simulink library "Feeder4_lib"  (Simulink 8.1)
settings: Solver=ode45  StartTime=0.0  StopTime=10.0  RelTol=1e-3
values from neighbouring files (symbols this model uses):
  DER_REL = xlsread('DER_relay.xlsx')    [relay_settings_init.m]
  Ts = 100E-6    (= 0.0001)    [BANSHEE_init.m]    (also in Ghost_init.m)
undefined symbols (not defined in the file or in its folder): CBID, Left, type, V
libraries: breaker_lib x9, Load_lib x7, cables_lib x3, relay_modbus_lib x3, rtio_generic_modbus x3, powerlib_meascontrol x3, NREL_Diesel_Genset_lib x2, BESS_lib x2, rtlab x2, simulink x2, ssn_lib x2, transformer_lib x1
settings Model: Creator=re25624  LastModifiedBy=MGC4

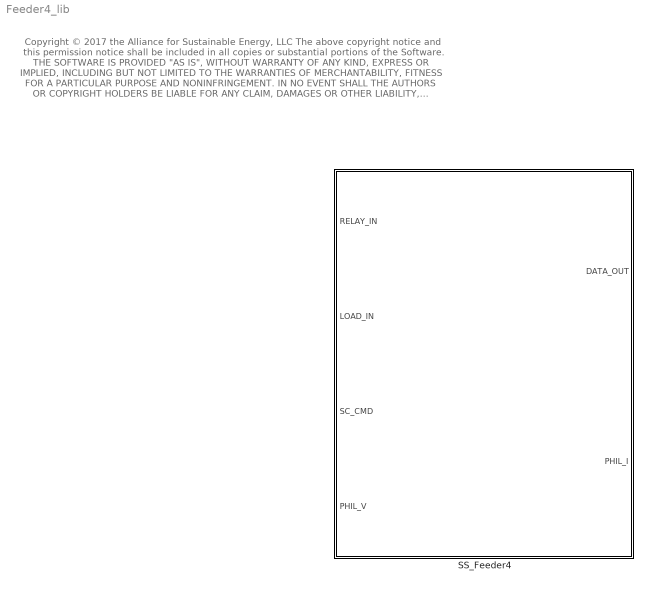
== system Feeder4_lib ==
  note: Copyright © 2017 the Alliance for Sustainable Energy, LLC
      |
      | The above copyright notice and this permission notice shall be included in all copies or substantial portions of the Software.
      |
      | THE SOFTWARE IS PROVIDED "AS IS", WITHOUT WARRANTY OF ANY KIND, EXPRESS OR IMPLIED, INCLUDING
      | BUT NOT LIMITED TO THE WARRANTIES OF MERCHANTABILITY, FITNESS FOR A PARTICULAR PURPOSE AND
      | NONINFRINGEMENT. IN NO EVENT SHALL THE AUTHORS OR COPYRIGHT HOLDERS BE LIABLE FOR ANY CLAIM,
      |  DAMAGES OR OTHER LIABILITY, WHETHER IN AN ACTION OF CONTRACT, TORT OR OTHERWISE, ARISING FROM,
      | OUT OF OR IN CONNECTION WITH THE SOFTWARE OR THE USE OR OTHER DEALINGS IN THE SOFTWARE
  SS_Feeder4 : Subsystem

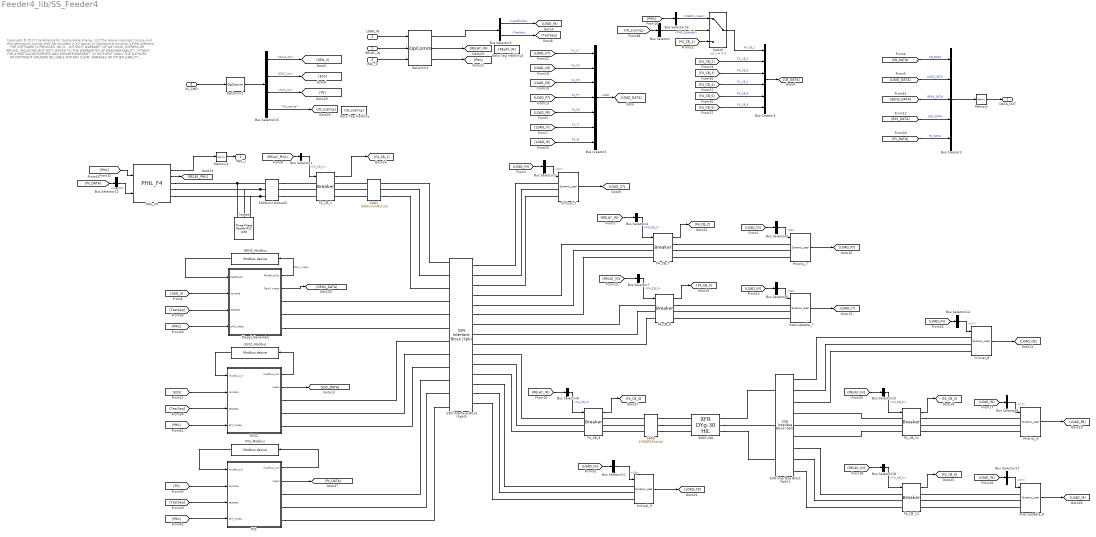
== system Feeder4_lib/SS_Feeder4 ==
  note: Copyright © 2017 the Alliance for Sustainable Energy, LLC
      |
      | The above copyright notice and this permission notice shall be included in all copies or substantial portions of the Software.
      |
      | THE SOFTWARE IS PROVIDED "AS IS", WITHOUT WARRANTY OF ANY KIND, EXPRESS OR IMPLIED, INCLUDING
      | BUT NOT LIMITED TO THE WARRANTIES OF MERCHANTABILITY, FITNESS FOR A PARTICULAR PURPOSE AND
      | NONINFRINGEMENT. IN NO EVENT SHALL THE AUTHORS OR COPYRIGHT HOLDERS BE LIABLE FOR ANY CLAIM,
      |  DAMAGES OR OTHER LIABILITY, WHETHER IN AN ACTION OF CONTRACT, TORT OR OTHERWISE, ARISING FROM,
      | OUT OF OR IN CONNECTION WITH THE SOFTWARE OR THE USE OR OTHER DEALINGS IN THE SOFTWARE
  RELAY_IN : Inport
  LOAD_IN : Inport  Port=2
  SC_CMD : Inport  Port=3
  PHIL_V : Inport  Port=4
  5000 kVA : transformer_lib/XFR DYg-30 HIL  Rating=50  Vp=480  Vs=208  Z=5.75  XR=4.7
  500kcmil-Mutual5 : cables_lib/500kcmil-Mutual  length=1000  par_sets=1  ratio=3
  Bus Creator2 : BusCreator  Inputs=5
  Bus Creator3 : BusCreator  Inputs=7
  Bus Creator5 : BusCreator  Inputs=6
  Bus Selector : BusSelector  OutputSignals=PHIL_Enabled
  Bus Selector1 : BusSelector  OutputSignals=F4_CB_1
  Bus Selector10 : BusSelector  OutputSignals=F4_CB_5
  Bus Selector11 : BusSelector  OutputSignals=C9
  Bus Selector12 : BusSelector  OutputSignals=pv_phil
  Bus Selector{2,9,14,17} (4 alike) : BusSelector  OutputSignals=C7
  Bus Selector15 : BusSelector  OutputSignals=Gen3_ctrl,ESS2_ctrl,PV2_ctrl,IO_scaling
  Bus Selector16 : BusSelector  OutputSignals=CB401_meas
  Bus Selector18 : BusSelector  OutputSignals=F4_CB_6
  Bus Selector3 : BusSelector  OutputSignals=C8
  Bus Selector4 : BusSelector  OutputSignals=F4_CB_2
  Bus Selector5 : BusSelector  OutputSignals=LoadProfile,TestSeq
  Bus Selector6 : BusSelector  OutputSignals=C8
  Bus Selector7 : BusSelector  OutputSignals=F4_CB_3
  Bus Selector8 : BusSelector  OutputSignals=F4_CB_4
  C401 : cables_lib/500kcmil-Mutual  length=2000  par_sets=1  ratio=3
  C403 : cables_lib/4//0AWG-Mutual  length=2000  par_sets=1  ratio=3
  Critical_7 : Load_lib/Dynamic_Load  V=480  kVA=25  PF=0.9  Ts=Ts
  Critical_8 : Load_lib/Dynamic_Load  V=208  kVA=20  PF=0.9  Ts=Ts
  Critical_9 : Load_lib/Dynamic_Load  V=480  kVA=3  PF=0.9  Ts=Ts
  Diesel_Generator : Subsystem
  ESS2 : Subsystem
  ESS2_Modbus : rtio_generic_modbus/Modbus device  conf_name=ESS2_modbus.opal  conf_name_mask=ESS2_modbus.xls  sample_time=Ts
  F4_CB_{1,7..9,11..12} (6 alike) : breaker_lib/Breaker  Ts=Ts  mech_delay=cb_mech_delay
  GEN3_Modbus : rtio_generic_modbus/Modbus device  conf_name=GEN3_modbus.opal  conf_name_mask=GEN3_modbus.xls  sample_time=Ts
  Goto Tag Visibility : GotoTagVisibility  GotoTag=IO_scaling
  Goto Tag Visibility2 : GotoTagVisibility  GotoTag=RELAY_IN
  Interruptable_7 : Load_lib/Dynamic_Load  V=480  kVA=30  PF=0.9  Ts=Ts
  Interruptable_8 : Load_lib/Dynamic_Load  V=208  kVA=20  PF=0.9  Ts=Ts
  Memory : Memory
  Memory1 : Memory
  OpComm1 : rtlab/OpComm  nbport=3  groupe_acq=1  subsys_rate=0  st=0  Synchronization=on  Interpolation=on  Threshold=1.0  Missed_Data=off  Sim_Time=off  Samples=off  dynSigOut=off  from_console=0  warning_done=off  writeOpCommFile=off  Offset=off
  OpComm2 : rtlab/OpComm  nbport=1  groupe_acq=1  subsys_rate=0  st=0  Synchronization=on  Interpolation=on  Threshold=1.0  Missed_Data=off  Sim_Time=off  Samples=off  dynSigOut=off  from_console=1  warning_done=off  writeOpCommFile=off  Offset=off
  PHIL_F4 : PHIL_lib/PHIL_F4
  PV2 : Subsystem
  PV2_Modbus : rtio_generic_modbus/Modbus device  conf_name=PV2_modbus.opal  conf_name_mask=PV2_modbus.xls  sample_time=Ts
  Priority_7 : Load_lib/Dynamic_Load  V=480  kVA=10  PF=0.9  Ts=Ts
  Priority_8 : Load_lib/Dynamic_Load  V=208  kVA=10  PF=0.9  Ts=Ts
  SSN Interface Block (3ph)1 : ssn_lib/SSN Interface Block (3ph)  nb_phase=3  nb_port=4  p1_type=V-type(Left)  p2_type=V-type (Right)  p3_type=V-type (Right)  p4_type=V-type (Right)  p5_type=V-type (Right)  p6_type=V-type (Right)  p7_type=V-type (Right)  p8_type=V-type(Left)  p9_type=V-type(Left)  p10_type=V-type(Left)  p11_type=V-type(Left)  p12_type=V-type(Left)  p13_type=V-type(Left)  p14_type=V-type(Left)  p15_type=V-type(Left)  p16_type=V-type(Left)  I_port_shunt_resistance=1e9
  SSN Interface Block (3ph)5 : ssn_lib/SSN Interface Block (3ph)  nb_phase=3  nb_port=9  p1_type=V-type(Left)  p2_type=V-type (Right)  p3_type=V-type (Right)  p4_type=V-type (Right)  p5_type=V-type (Right)  p6_type=V-type (Right)  p7_type=V-type(Left)  p8_type=V-type(Left)  p9_type=V-type(Left)  p10_type=V-type(Left)  p11_type=V-type(Left)  p12_type=V-type(Left)  p13_type=V-type(Left)  p14_type=V-type(Left)  p15_type=V-type(Left)  p16_type=V-type(Left)  I_port_shunt_resistance=1e9
  Switch : Switch  Threshold=0.5
  losses : powerlib/Elements/Three-Phase Parallel RLC Load  LConnTagsString=A|B|C  Configuration=Y (grounded)  NominalVoltage=480  NominalFrequency=60  ActivePower=1e3  InductivePower=1e3  CapacitivePower=0  Measurements=None  LoadType=constant Z
  DATA_OUT : Outport
  PHIL_I : Outport  Port=2
  tag scope: IO_scaling=scoped, RELAY_IN=scoped
  wires:
  Bus Selector12/1 -> PHIL_F4/2  "<pv_phil>"
  [PV_DATA] -> Bus Selector12/1
  [PHIL] -> PV2/4(phil_meas)
  [PHIL] -> ESS2/4(phil_meas)
  [PHIL] -> Diesel_Generator/4(phil_meas)
  [TestSeq] -> Diesel_Generator/3(testseq)
  [TestSeq] -> ESS2/3(testseq)
  [PV] -> PV2/2(console)
  [TestSeq] -> PV2/3(testseq)
  [PHIL] -> PHIL_F4/1
  [F4_CB_1] -> Switch/3
  [PHIL] -> Bus Selector16/1
  Bus Selector/1 -> Switch/2  "<PHIL_Enabled>"
  [IO_scaling] -> Bus Selector/1
  Bus Selector16/1 -> Switch/1  "<CB401_meas>"
  Bus Selector1/1 -> F4_CB_1/1  "<F4_CB_1>"
  [RELAY_PHIL] -> Bus Selector1/1
  PHIL_F4/2 -> [RELAY_PHIL]
  PHIL_F4/1 -> Memory1/1
  Bus Selector15/4 -> [IO_scaling]  "<IO_scaling>"
  Bus Selector5/2 -> [TestSeq]  "<TestSeq>"
  Bus Selector5/1 -> [LOAD_IN]  "<LoadProfile>"
  OpComm1/1 -> Bus Selector5/1
  OpComm1/3 -> [PHIL]
  PHIL_V/1 -> OpComm1/3
  Memory1/1 -> PHIL_I/1
  [LOAD_I8] -> Bus Creator3/7  "F4_I8"
  [LOAD_P8] -> Bus Creator3/5  "F4_P8"
  [LOAD_P7] -> Bus Creator3/4  "F4_P7"
  [LOAD_I7] -> Bus Creator3/6  "F4_I7"
  Diesel_Generator/2(Gen3 meas) -> [GEN3_DATA]
  Diesel_Generator/1(ModbusOut) -> GEN3_Modbus/1  "Gen_meas"
  GEN3_Modbus/1 -> Diesel_Generator/1(ModbusIn)
  ESS2_Modbus/1 -> ESS2/1(modbus_in)
  ESS2/1(modbus_out) -> ESS2_Modbus/1
  ESS2/2(meas) -> [ESS_DATA]
  PV2/2(meas) -> [PV_DATA]
  PV2/1(modbus_out) -> PV2_Modbus/1
  PV2_Modbus/1 -> PV2/1(modbus_in)
  Bus Selector15/3 -> [PV]  "<PV2_ctrl>"
  [PV_DATA] -> Bus Creator2/5  "PV_DATA"
  F4_CB_12/1 -> [F4_CB_6]
  Bus Selector18/1 -> F4_CB_12/1  "<F4_CB_6>"
  [RELAY_IN] -> Bus Selector18/1
  [LOAD_IN] -> Bus Selector17/1
  Bus Selector17/1 -> Interruptable_8/1  "<C7>"
  Interruptable_8/1 -> [LOAD_I8]
  [LOAD_IN] -> Bus Selector14/1
  Bus Selector14/1 -> Critical_8/1  "<C7>"
  Critical_8/1 -> [LOAD_C8]
  F4_CB_11/1 -> [F4_CB_5]
  Bus Selector10/1 -> F4_CB_11/1  "<F4_CB_5>"
  [RELAY_IN] -> Bus Selector10/1
  [LOAD_IN] -> Bus Selector9/1
  Bus Selector9/1 -> Priority_8/1  "<C7>"
  Priority_8/1 -> [LOAD_P8]
  F4_CB_9/1 -> [F4_CB_4]
  Bus Selector8/1 -> F4_CB_9/1  "<F4_CB_4>"
  [RELAY_IN] -> Bus Selector8/1
  F4_CB_8/1 -> [F4_CB_3]
  Bus Selector7/1 -> F4_CB_8/1  "<F4_CB_3>"
  [RELAY_IN] -> Bus Selector7/1
  [LOAD_IN] -> Bus Selector6/1
  Bus Selector6/1 -> Interruptable_7/1  "<C8>"
  Interruptable_7/1 -> [LOAD_I7]
  [ESS] -> ESS2/2(console)
  [ESS_DATA] -> Bus Creator2/4  "ESS_DATA"
  Bus Selector15/2 -> [ESS]  "<ESS2_ctrl>"
  [GEN_3] -> Diesel_Generator/2(console)
  F4_CB_7/1 -> [F4_CB_2]
  Bus Selector4/1 -> F4_CB_7/1  "<F4_CB_2>"
  [RELAY_IN] -> Bus Selector4/1
  [LOAD_IN] -> Bus Selector3/1
  Bus Selector3/1 -> Priority_7/1  "<C8>"
  Priority_7/1 -> [LOAD_P7]
  [LOAD_IN] -> Bus Selector2/1
  Bus Selector2/1 -> Critical_7/1  "<C7>"
  Critical_7/1 -> [LOAD_C7]
  [LOAD_IN] -> Bus Selector11/1
  Bus Selector11/1 -> Critical_9/1  "<C9>"
  Critical_9/1 -> [LOAD_C9]
  LOAD_IN/1 -> OpComm1/1
  [LOAD_C8] -> Bus Creator3/2  "F4_C8"
  [LOAD_C7] -> Bus Creator3/1  "F4_C7"
  [LOAD_C9] -> Bus Creator3/3  "F4_C9"
  Bus Creator3/1 -> [LOAD_DATA]  "LOAD"
  Switch/1 -> Bus Creator5/1  "F4_CB_1"
  [F4_CB_5] -> Bus Creator5/5  "F4_CB_5"
  [F4_CB_6] -> Bus Creator5/6  "F4_CB_6"
  [F4_CB_3] -> Bus Creator5/3  "F4_CB_3"
  [F4_CB_2] -> Bus Creator5/2  "F4_CB_2"
  [F4_CB_4] -> Bus Creator5/4  "F4_CB_4"
  Bus Creator5/1 -> [CB_DATA]
  RELAY_IN/1 -> OpComm1/2
  OpComm1/2 -> [RELAY_IN]
  F4_CB_1/1 -> [F4_CB_1]
  SC_CMD/1 -> OpComm2/1
  Memory/1 -> DATA_OUT/1
  OpComm2/1 -> Bus Selector15/1
  Bus Creator2/1 -> Memory/1
  [CB_DATA] -> Bus Creator2/1  "CB_DATA"
  [LOAD_DATA] -> Bus Creator2/2  "LOAD_DATA"
  [GEN3_DATA] -> Bus Creator2/3  "GEN3_DATA"
  Bus Selector15/1 -> [GEN_3]  "<Gen3_ctrl>"
  connections:
  SSN Interface Block (3ph)5/RConn13 -- Critical_9/LConn1
  SSN Interface Block (3ph)5/RConn14 -- Critical_9/LConn2
  SSN Interface Block (3ph)5/RConn15 -- Critical_9/LConn3
  PV2/RConn3 -- SSN Interface Block (3ph)5/LConn12
  PV2/RConn2 -- SSN Interface Block (3ph)5/LConn11
  PV2/RConn1 -- SSN Interface Block (3ph)5/LConn10
  ESS2/RConn2 -- SSN Interface Block (3ph)5/LConn8
  ESS2/RConn1 -- SSN Interface Block (3ph)5/LConn7
  ESS2/RConn3 -- SSN Interface Block (3ph)5/LConn9
  Diesel_Generator/RConn3 -- SSN Interface Block (3ph)5/LConn6
  Diesel_Generator/RConn2 -- SSN Interface Block (3ph)5/LConn5
  Diesel_Generator/RConn1 -- SSN Interface Block (3ph)5/LConn4
  SSN Interface Block (3ph)1/RConn7 -- F4_CB_12/LConn1
  SSN Interface Block (3ph)1/RConn8 -- F4_CB_12/LConn2
  SSN Interface Block (3ph)1/RConn9 -- F4_CB_12/LConn3
  F4_CB_11/LConn1 -- SSN Interface Block (3ph)1/RConn4
  F4_CB_11/LConn2 -- SSN Interface Block (3ph)1/RConn5
  F4_CB_11/LConn3 -- SSN Interface Block (3ph)1/RConn6
  SSN Interface Block (3ph)1/RConn1 -- Critical_8/LConn1
  SSN Interface Block (3ph)1/RConn2 -- Critical_8/LConn2
  SSN Interface Block (3ph)1/RConn3 -- Critical_8/LConn3
  F4_CB_12/RConn2 -- Interruptable_8/LConn2
  Interruptable_8/LConn3 -- F4_CB_12/RConn3
  Interruptable_8/LConn1 -- F4_CB_12/RConn1
  F4_CB_11/RConn3 -- Priority_8/LConn3
  F4_CB_11/RConn1 -- Priority_8/LConn1
  Priority_8/LConn2 -- F4_CB_11/RConn2
  5000 kVA/RConn1 -- SSN Interface Block (3ph)1/LConn1
  5000 kVA/RConn3 -- SSN Interface Block (3ph)1/LConn3
  5000 kVA/RConn2 -- SSN Interface Block (3ph)1/LConn2
  C403/RConn3 -- 5000 kVA/LConn3
  C403/RConn1 -- 5000 kVA/LConn1
  C403/RConn2 -- 5000 kVA/LConn2
  F4_CB_9/LConn2 -- SSN Interface Block (3ph)5/RConn11
  F4_CB_9/LConn1 -- SSN Interface Block (3ph)5/RConn10
  F4_CB_9/LConn3 -- SSN Interface Block (3ph)5/RConn12
  C403/LConn2 -- F4_CB_9/RConn2
  C403/LConn3 -- F4_CB_9/RConn3
  C403/LConn1 -- F4_CB_9/RConn1
  Interruptable_7/LConn2 -- F4_CB_8/RConn2
  F4_CB_8/RConn3 -- Interruptable_7/LConn3
  F4_CB_8/RConn1 -- Interruptable_7/LConn1
  F4_CB_8/LConn3 -- SSN Interface Block (3ph)5/RConn9
  F4_CB_8/LConn2 -- SSN Interface Block (3ph)5/RConn8
  F4_CB_8/LConn1 -- SSN Interface Block (3ph)5/RConn7
  SSN Interface Block (3ph)5/RConn2 -- Critical_7/LConn2
  SSN Interface Block (3ph)5/RConn3 -- Critical_7/LConn3
  SSN Interface Block (3ph)5/RConn1 -- Critical_7/LConn1
  SSN Interface Block (3ph)5/RConn4 -- F4_CB_7/LConn1
  SSN Interface Block (3ph)5/RConn5 -- F4_CB_7/LConn2
  SSN Interface Block (3ph)5/RConn6 -- F4_CB_7/LConn3
  F4_CB_7/RConn1 -- Priority_7/LConn1
  F4_CB_7/RConn3 -- Priority_7/LConn3
  F4_CB_7/RConn2 -- Priority_7/LConn2
  C401/LConn3 -- F4_CB_1/RConn3
  C401/LConn1 -- F4_CB_1/RConn1
  C401/LConn2 -- F4_CB_1/RConn2
  500kcmil-Mutual5/RConn1 -- F4_CB_1/LConn1
  500kcmil-Mutual5/RConn2 -- F4_CB_1/LConn2
  500kcmil-Mutual5/RConn3 -- F4_CB_1/LConn3
  C401/RConn1 -- SSN Interface Block (3ph)5/LConn1
  C401/RConn2 -- SSN Interface Block (3ph)5/LConn2
  C401/RConn3 -- SSN Interface Block (3ph)5/LConn3
  losses/LConn1 -- PHIL_F4/RConn1 -- 500kcmil-Mutual5/LConn1
  500kcmil-Mutual5/LConn2 -- PHIL_F4/RConn2 -- losses/LConn2
  500kcmil-Mutual5/LConn3 -- PHIL_F4/RConn3 -- losses/LConn3

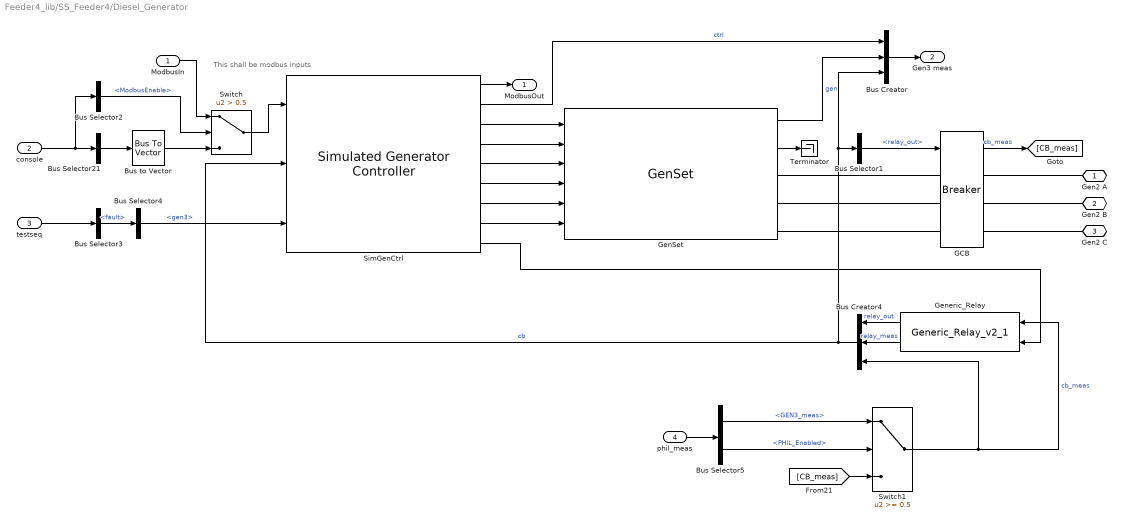
== system Feeder4_lib/SS_Feeder4/Diesel_Generator ==
  note: This shall be modbus inputs
  ModbusIn : Inport
  console : Inport  Port=2
  testseq : Inport  Port=3
  phil_meas : Inport  Port=4
  Bus Creator : BusCreator  Inputs=3
  Bus Creator4 : BusCreator  Inputs=3
  Bus Selector1 : BusSelector  OutputSignals=relay_out
  Bus Selector2 : BusSelector  OutputSignals=ModbusEnable
  Bus Selector21 : BusSelector  OutputSignals=ModbusFromSC.Ctrl,ModbusFromSC.PCmd,ModbusFromSC.QCmd,ModbusFromSC.VoltCmd,ModbusFromSC.FreqCmd,ModbusFromSC.signal6,ModbusFromSC.signal7,ModbusFromSC.signal8  OutputAsBus=on
  Bus Selector3 : BusSelector  OutputSignals=fault
  Bus Selector4 : BusSelector  OutputSignals=gen3
  Bus Selector5 : BusSelector  OutputSignals=GEN3_meas,PHIL_Enabled
  Bus to Vector : BusToVector
  GCB : breaker_lib/Breaker  Ts=Ts  mech_delay=cb_mech_delay
  GenSet : NREL_Diesel_Genset_lib/GenSet  GenSel=80kVA diesel generator
  Generic_Relay : relay_modbus_lib/Generic_Relay_v2_1  Ts=Ts  relay_settings=[DER_REL(CBID.GEN3,:)]
  SimGenCtrl : NREL_Diesel_Genset_lib/Simulated Generator Controller  GenSel=80kVA diesel generator
  Switch : Switch  Criteria=u2 > Threshold  Threshold=0.5
  Switch1 : Switch  Threshold=0.5
  Terminator : Terminator
  Gen2 A : PMIOPort  Port=1  Side=Right
  Gen2 B : PMIOPort  Port=2  Side=Right
  Gen2 C : PMIOPort  Port=3  Side=Right
  ModbusOut : Outport
  Gen3 meas : Outport  Port=2
  wires:
  Bus Selector1/1 -> GCB/1  "<relay_out>"
  Switch1/1 -> Generic_Relay/1, Bus Creator4/3  "cb_meas"
  GCB/1 -> [CB_meas]  "cb_meas"
  Bus Selector5/2 -> Switch1/2  "<PHIL_Enabled>"
  Bus Selector5/1 -> Switch1/1  "<GEN3_meas>"
  [CB_meas] -> Switch1/3
  phil_meas/1 -> Bus Selector5/1
  Bus Selector4/1 -> SimGenCtrl/3  "<gen3>"
  Bus Selector3/1 -> Bus Selector4/1  "<fault>"
  testseq/1 -> Bus Selector3/1
  SimGenCtrl/9 -> Generic_Relay/2
  SimGenCtrl/1 -> ModbusOut/1
  SimGenCtrl/8 -> GenSet/6
  SimGenCtrl/7 -> GenSet/5
  SimGenCtrl/3 -> GenSet/1
  SimGenCtrl/4 -> GenSet/2
  SimGenCtrl/5 -> GenSet/3
  SimGenCtrl/6 -> GenSet/4
  GenSet/1 -> Bus Creator/2  "gen"
  Bus Creator4/1 -> Bus Creator/3, Bus Selector1/1, SimGenCtrl/2  "cb"
  console/1 -> Bus Selector21/1, Bus Selector2/1
  Bus Selector2/1 -> Switch/2  "<ModbusEnable>"
  ModbusIn/1 -> Switch/1
  Bus Selector21/1 -> Bus to Vector/1
  Bus to Vector/1 -> Switch/3
  Switch/1 -> SimGenCtrl/1
  Generic_Relay/1 -> Bus Creator4/1  "relay_out"
  Generic_Relay/2 -> Bus Creator4/2  "relay_meas"
  Bus Creator/1 -> Gen3 meas/1
  SimGenCtrl/2 -> Bus Creator/1  "ctrl"
  GenSet/2 -> Terminator/1
  connections:
  Gen2 A/RConn1 -- GCB/RConn1
  GCB/RConn2 -- Gen2 B/RConn1
  Gen2 C/RConn1 -- GCB/RConn3
  GenSet/RConn1 -- GCB/LConn1
  GenSet/RConn2 -- GCB/LConn2
  GenSet/RConn3 -- GCB/LConn3

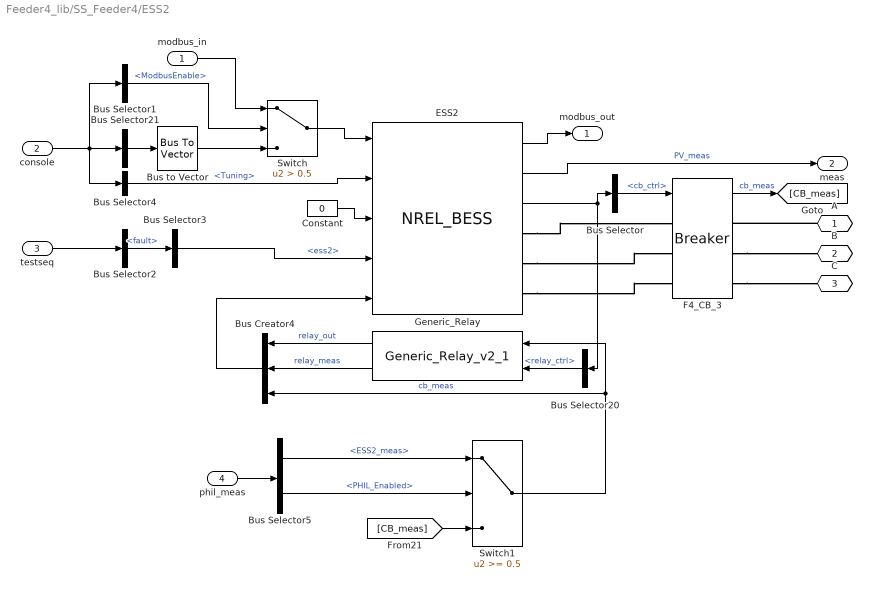
== system Feeder4_lib/SS_Feeder4/ESS2 ==
  modbus_in : Inport
  console : Inport  Port=2
  testseq : Inport  Port=3
  phil_meas : Inport  Port=4
  Bus Creator4 : BusCreator  Inputs=3
  Bus Selector : BusSelector  OutputSignals=cb_ctrl
  Bus Selector1 : BusSelector  OutputSignals=ModbusEnable
  Bus Selector2 : BusSelector  OutputSignals=fault
  Bus Selector20 : BusSelector  OutputSignals=relay_ctrl
  Bus Selector21 : BusSelector  OutputSignals=ModbusFromSC.Ctrl,ModbusFromSC.PCmd,ModbusFromSC.QCmd,ModbusFromSC.VoltCmd,ModbusFromSC.FreqCmd,ModbusFromSC.signal6,ModbusFromSC.signal7,ModbusFromSC.signal8  OutputAsBus=on
  Bus Selector3 : BusSelector  OutputSignals=ess2
  Bus Selector4 : BusSelector  OutputSignals=Tuning
  Bus Selector5 : BusSelector  OutputSignals=ESS2_meas,PHIL_Enabled
  Bus to Vector : BusToVector
  Constant : Constant  Value=0
  ESS2 : BESS_lib/NREL_BESS  InvType=ESS Inverter  Sn=250  Vn=480  b_Vdc_nom=1000  b_kWh=600  b_esr=0.1  r_I_max=3  Tc=Ts  MbusPrecInc=on  ExtTuningEna=on
  F4_CB_3 : breaker_lib/Breaker  Ts=Ts  mech_delay=cb_mech_delay
  Generic_Relay : relay_modbus_lib/Generic_Relay_v2_1  Ts=Ts  relay_settings=[DER_REL(CBID.ESS2,:)]
  Switch : Switch  Criteria=u2 > Threshold  Threshold=0.5
  Switch1 : Switch  Threshold=0.5
  A : PMIOPort  Port=1  Side=Right
  B : PMIOPort  Port=2  Side=Right
  C : PMIOPort  Port=3  Side=Right
  modbus_out : Outport
  meas : Outport  Port=2
  wires:
  Bus Selector4/1 -> ESS2/2  "<Tuning>"
  Bus Selector/1 -> F4_CB_3/1  "<cb_ctrl>"
  F4_CB_3/1 -> [CB_meas]  "cb_meas"
  Switch1/1 -> Bus Creator4/3, Generic_Relay/1  "cb_meas"
  Bus Selector5/2 -> Switch1/2  "<PHIL_Enabled>"
  Bus Selector5/1 -> Switch1/1  "<ESS2_meas>"
  [CB_meas] -> Switch1/3
  phil_meas/1 -> Bus Selector5/1
  Bus Selector3/1 -> ESS2/4  "<ess2>"
  Bus Selector2/1 -> Bus Selector3/1  "<fault>"
  testseq/1 -> Bus Selector2/1
  Constant/1 -> ESS2/3
  Bus to Vector/1 -> Switch/3
  ESS2/3 -> Bus Selector20/1, Bus Selector/1
  Switch/1 -> ESS2/1
  Bus Selector21/1 -> Bus to Vector/1
  modbus_in/1 -> Switch/1
  ESS2/1 -> modbus_out/1
  Bus Selector1/1 -> Switch/2  "<ModbusEnable>"
  console/1 -> Bus Selector21/1, Bus Selector1/1, Bus Selector4/1
  Bus Selector20/1 -> Generic_Relay/2  "<relay_ctrl>"
  Generic_Relay/1 -> Bus Creator4/1  "relay_out"
  ESS2/2 -> meas/1  "PV_meas"
  Generic_Relay/2 -> Bus Creator4/2  "relay_meas"
  Bus Creator4/1 -> ESS2/5
  connections:
  F4_CB_3/RConn3 -- C/RConn1
  A/RConn1 -- F4_CB_3/RConn1
  ESS2/RConn1 -- F4_CB_3/LConn1
  ESS2/RConn3 -- F4_CB_3/LConn3
  ESS2/RConn2 -- F4_CB_3/LConn2
  F4_CB_3/RConn2 -- B/RConn1

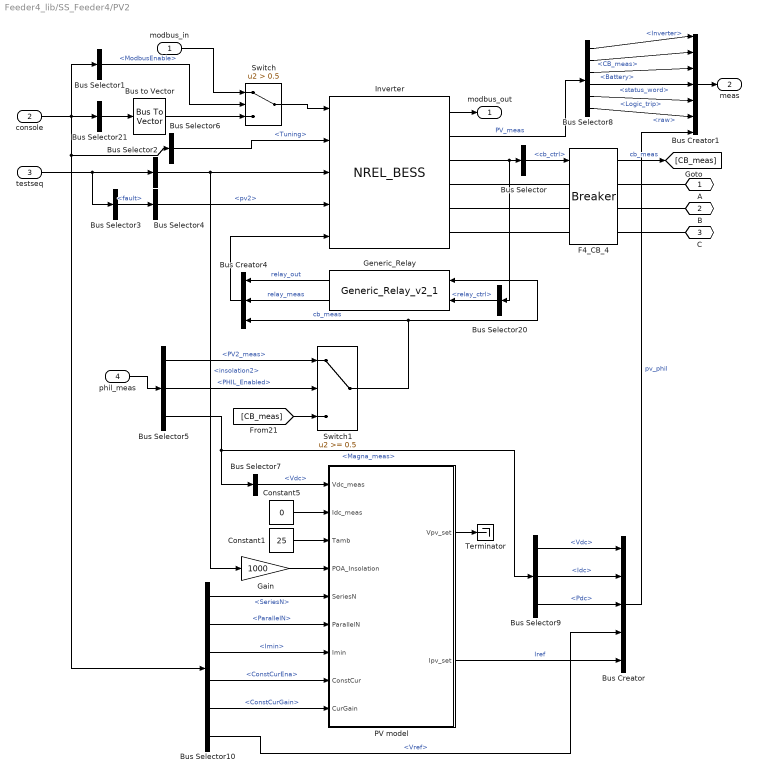
== system Feeder4_lib/SS_Feeder4/PV2 ==
  modbus_in : Inport
  console : Inport  Port=2
  testseq : Inport  Port=3
  phil_meas : Inport  Port=4
  Bus Creator : BusCreator  Inputs=5
  Bus Creator1 : BusCreator  Inputs=7
  Bus Creator4 : BusCreator  Inputs=3
  Bus Selector : BusSelector  OutputSignals=cb_ctrl
  Bus Selector1 : BusSelector  OutputSignals=ModbusEnable
  Bus Selector10 : BusSelector  OutputSignals=Tuning.SeriesN,Tuning.ParallelN,Tuning.Imin,Tuning.ConstCurEna,Tuning.ConstCurGain,Tuning.Vref
  Bus Selector2 : BusSelector  OutputSignals=pv.insolation2
  Bus Selector20 : BusSelector  OutputSignals=relay_ctrl
  Bus Selector21 : BusSelector  OutputSignals=ModbusFromSC.Ctrl,ModbusFromSC.PCmd,ModbusFromSC.QCmd,ModbusFromSC.VoltCmd,ModbusFromSC.FreqCmd,ModbusFromSC.signal6,ModbusFromSC.signal7,ModbusFromSC.signal8  OutputAsBus=on
  Bus Selector3 : BusSelector  OutputSignals=fault
  Bus Selector4 : BusSelector  OutputSignals=pv2
  Bus Selector5 : BusSelector  OutputSignals=PV2_meas,PHIL_Enabled,Magna_meas
  Bus Selector6 : BusSelector  OutputSignals=Tuning
  Bus Selector7 : BusSelector  OutputSignals=Vdc
  Bus Selector8 : BusSelector  OutputSignals=Inverter,CB_meas,Battery,status_word,Logic_trip,raw
  Bus Selector9 : BusSelector  OutputSignals=Vdc,Idc,Pdc
  Bus to Vector : BusToVector
  Constant1 : Constant  Value=25
  Constant5 : Constant  Value=0
  F4_CB_4 : breaker_lib/Breaker  Ts=Ts  mech_delay=cb_mech_delay
  Gain : Gain  Gain=1000
  Generic_Relay : relay_modbus_lib/Generic_Relay_v2_1  Ts=Ts  relay_settings=[DER_REL(CBID.PV2,:)]
  Inverter : BESS_lib/NREL_BESS  InvType=PV Inverter  Sn=100  Vn=480  b_Vdc_nom=1000  b_kWh=1  b_esr=0.1  r_I_max=1.2  Tc=Ts  MbusPrecInc=on  ExtTuningEna=on
  PV model : Subsystem
  Switch : Switch  Criteria=u2 > Threshold  Threshold=0.5
  Switch1 : Switch  Threshold=0.5
  Terminator : Terminator
  A : PMIOPort  Port=1  Side=Right
  B : PMIOPort  Port=2  Side=Right
  C : PMIOPort  Port=3  Side=Right
  modbus_out : Outport
  meas : Outport  Port=2
  wires:
  Bus Selector10/4 -> PV model/8(ConstCur)  "<ConstCurEna>"
  Bus Selector10/5 -> PV model/9(CurGain)  "<ConstCurGain>"
  PV model/2(Ipv_set) -> Bus Creator/5  "Iref"
  Bus Selector10/6 -> Bus Creator/4  "<Vref>"
  Bus Selector10/3 -> PV model/7(Imin)  "<Imin>"
  Bus Selector10/2 -> PV model/6(ParallelN)  "<ParallelN>"
  Bus Selector10/1 -> PV model/5(SeriesN)  "<SeriesN>"
  Bus Selector9/1 -> Bus Creator/1  "<Vdc>"
  Bus Selector9/3 -> Bus Creator/3  "<Pdc>"
  Bus Selector9/2 -> Bus Creator/2  "<Idc>"
  Bus Creator1/1 -> meas/1
  Bus Selector8/1 -> Bus Creator1/1  "<Inverter>"
  Bus Selector8/2 -> Bus Creator1/2  "<CB_meas>"
  Bus Selector8/3 -> Bus Creator1/3  "<Battery>"
  Bus Selector8/4 -> Bus Creator1/4  "<status_word>"
  Bus Selector8/5 -> Bus Creator1/5  "<Logic_trip>"
  Bus Selector8/6 -> Bus Creator1/6  "<raw>"
  Bus Creator/1 -> Bus Creator1/7  "pv_phil"
  PV model/1(Vpv_set) -> Terminator/1
  Bus Selector7/1 -> PV model/1(Vdc_meas)  "<Vdc>"
  Bus Selector5/3 -> Bus Selector7/1, Bus Selector9/1  "<Magna_meas>"
  Gain/1 -> PV model/4(POA_Insolation)
  Constant5/1 -> PV model/2(Idc_meas)
  Constant1/1 -> PV model/3(Tamb)
  Bus Selector6/1 -> Inverter/2  "<Tuning>"
  Bus Selector/1 -> F4_CB_4/1  "<cb_ctrl>"
  F4_CB_4/1 -> [CB_meas]  "cb_meas"
  Switch1/1 -> Generic_Relay/1, Bus Creator4/3  "cb_meas"
  Bus Selector5/2 -> Switch1/2  "<PHIL_Enabled>"
  Bus Selector5/1 -> Switch1/1  "<PV2_meas>"
  [CB_meas] -> Switch1/3
  phil_meas/1 -> Bus Selector5/1
  Bus Selector4/1 -> Inverter/4  "<pv2>"
  Bus Selector3/1 -> Bus Selector4/1  "<fault>"
  Bus Selector2/1 -> Inverter/3, Gain/1  "<insolation2>"
  Bus Selector21/1 -> Bus to Vector/1
  Bus Selector1/1 -> Switch/2  "<ModbusEnable>"
  console/1 -> Bus Selector1/1, Bus Selector21/1, Bus Selector10/1, Bus Selector6/1
  testseq/1 -> Bus Selector2/1, Bus Selector3/1
  Bus Creator4/1 -> Inverter/5
  Generic_Relay/2 -> Bus Creator4/2  "relay_meas"
  Inverter/2 -> Bus Selector8/1  "PV_meas"
  Generic_Relay/1 -> Bus Creator4/1  "relay_out"
  Bus Selector20/1 -> Generic_Relay/2  "<relay_ctrl>"
  Inverter/1 -> modbus_out/1
  modbus_in/1 -> Switch/1
  Bus to Vector/1 -> Switch/3
  Switch/1 -> Inverter/1
  Inverter/3 -> Bus Selector/1, Bus Selector20/1
  connections:
  F4_CB_4/RConn2 -- B/RConn1
  Inverter/RConn2 -- F4_CB_4/LConn2
  Inverter/RConn3 -- F4_CB_4/LConn3
  Inverter/RConn1 -- F4_CB_4/LConn1
  A/RConn1 -- F4_CB_4/RConn1
  F4_CB_4/RConn3 -- C/RConn1

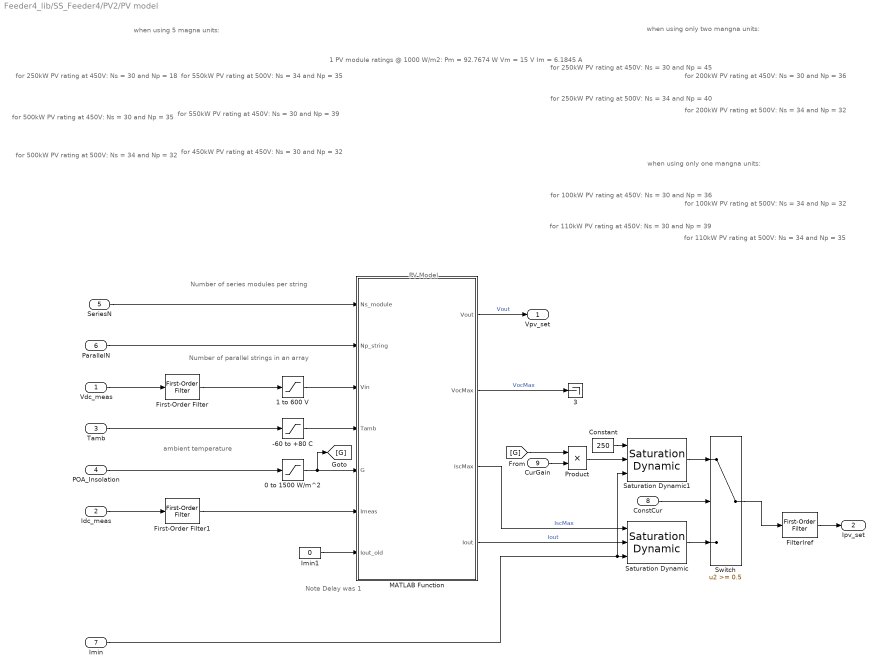
== system Feeder4_lib/SS_Feeder4/PV2/PV model ==
  note: for 110kW PV rating at 500V:
      | Ns = 34 and Np = 35
  note: for 100kW PV rating at 500V:
      | Ns = 34 and Np = 32
  note: for 100kW PV rating at 450V:
      | Ns = 30 and Np = 36
  note: for 110kW PV rating at 450V:
      | Ns = 30 and Np = 39
  note: when using only one mangna units:
  note: for 200kW PV rating at 500V:
      | Ns = 34 and Np = 32
  note: for 200kW PV rating at 450V:
      | Ns = 30 and Np = 36
  note: for 250kW PV rating at 450V:
      | Ns = 30 and Np = 45
  note: when using 5 magna units:
  note: for 250kW PV rating at 500V:
      | Ns = 34 and Np = 40
  note: when using only two mangna units:
  note: for 550kW PV rating at 500V:
      | Ns = 34 and Np = 35
  note: 1 PV module ratings @ 1000 W/m2:
      | Pm = 92.7674 W
      | Vm = 15 V
      | Im = 6.1845 A
  note: for 500kW PV rating at 500V:
      | Ns = 34 and Np = 32
  note: for 450kW PV rating at 450V:
      | Ns = 30 and Np = 32
  note: for 550kW PV rating at 450V:
      | Ns = 30 and Np = 39
  note: for 250kW PV rating at 450V:
      | Ns = 30 and Np = 18
  note: for 500kW PV rating at 450V:
      | Ns = 30 and Np = 35
  note: ambient temperature
  note: Number of parallel strings in an array
  note: Number of series modules per string
  note: Note Delay was 1
  note: PV Model
  Vdc_meas : Inport
  Idc_meas : Inport  Port=2
  Tamb : Inport  Port=3
  POA_Insolation : Inport  Port=4
  SeriesN : Inport  Port=5
  ParallelN : Inport  Port=6
  Imin : Inport  Port=7
  ConstCur : Inport  Port=8
  CurGain : Inport  Port=9
  " 3" : Terminator
  -60 to +80 C : Saturate  UpperLimit=80  LowerLimit=-60
  0 to 1500 W/m^2 : Saturate  UpperLimit=1500  LowerLimit=0
  1 to 600 V : Saturate  UpperLimit=600  LowerLimit=1
  Constant : Constant  Value=250
  FilterIref : powerlib_meascontrol/Filters/First-Order Filter  FilterType=Lowpass  Tc=10e-3  Ts=Ts  Initialize=on  Vac_Init=[0, 0, 60]  Vdc_Init=0  PlotResponse=off  FreqRange="[0,  200,  1]"
      settings: AttributesFormatString=%<Tc>
  First-Order Filter : powerlib_meascontrol/Filters/First-Order Filter  FilterType=Lowpass  Tc=200e-3  Ts=100e-6  Initialize=on  Vac_Init=[0, 0, 60]  Vdc_Init=0  PlotResponse=off  FreqRange="[0,  200,  1]"
  First-Order Filter1 : powerlib_meascontrol/Filters/First-Order Filter  FilterType=Lowpass  Tc=200e-3  Ts=100e-6  Initialize=on  Vac_Init=[0, 0, 60]  Vdc_Init=0  PlotResponse=off  FreqRange="[0,  200,  1]"
  Imin1 : Constant  Value=0
  MATLAB Function : MATLAB Function  TreatAsAtomicUnit=on
  Product : Product
  Saturation Dynamic : simulink/Discontinuities/Saturation Dynamic  OutMin=[]  OutMax=[]  OutDataTypeStr=Inherit: Same as second input  OutDataType=fixdt(1, 16)  OutScaling=2^-10  DoSatur=off
  Saturation Dynamic1 : simulink/Discontinuities/Saturation Dynamic  OutMin=[]  OutMax=[]  OutDataTypeStr=Inherit: Same as second input  OutDataType=fixdt(1, 16)  OutScaling=2^-10  DoSatur=off
  Switch : Switch  Threshold=0.5
  Vpv_set : Outport
  Ipv_set : Outport  Port=2
  wires:
  Constant/1 -> Saturation Dynamic1/1
  Saturation Dynamic1/1 -> Switch/1
  Product/1 -> Saturation Dynamic1/2
  [G] -> Product/1
  CurGain/1 -> Product/2
  FilterIref/1 -> Ipv_set/1
  ConstCur/1 -> Switch/2
  Switch/1 -> FilterIref/1
  MATLAB Function/1(Vout) -> Vpv_set/1  "Vout"
  MATLAB Function/2(VocMax) -> " 3"/1  "VocMax"
  MATLAB Function/3(IscMax) -> Saturation Dynamic/1  "IscMax"
  Imin/1 -> Saturation Dynamic/3, Saturation Dynamic1/3
  MATLAB Function/4(Iout) -> Saturation Dynamic/2  "Iout"
  First-Order Filter1/1 -> MATLAB Function/6(Imeas)
  First-Order Filter/1 -> 1 to 600 V/1
  Idc_meas/1 -> First-Order Filter1/1
  1 to 600 V/1 -> MATLAB Function/3(Vin)
  -60 to +80 C/1 -> MATLAB Function/4(Tamb)
  0 to 1500 W/m^2/1 -> MATLAB Function/5(G), [G]
  Saturation Dynamic/1 -> Switch/3
  Vdc_meas/1 -> First-Order Filter/1
  POA_Insolation/1 -> 0 to 1500 W/m^2/1
  Tamb/1 -> -60 to +80 C/1
  ParallelN/1 -> MATLAB Function/2(Np_string)
  SeriesN/1 -> MATLAB Function/1(Ns_module)
  Imin1/1 -> MATLAB Function/7(Iout_old)

== matlab function SS_Feeder4/PV2/PV model/MATLAB Function ==
  data: Ns_module input double; Vout output double; VocMax output double; IscMax output double; Np_string input double; Vin input double; Tamb input double; G input double; Imeas input double; Iout_old input double; Iout output double
function [Vout, VocMax, IscMax, Iout]  = bp_sx110(Ns_module, Np_string, Vin, Tamb, G, Imeas, Iout_old)
%
% function bp_sx110.m models the BP SX 110 PV module
%	module date found at: http://www.posharp.com/bp-sx110-solar-panel-from-bp-solar_p60866579d.aspx
%
% P.S.: according to: https://www.homepower.com/view/?file=HP113_pg106_WordPower
%	PV array ---> set of parallel and series modules
%	PV module (sometimes called panel) ---> set of parallel and series PV cells
%	PV string ---> set of series connected modules (panels)
%
% The function calculates array output current under given:
%	1- number of modules in series (modules in a string)
%	2- number of strings in parallel
%	3- irradiance and temperature
%
% This model was written by Noel Dillman and Blake Lundstrom of the Colorado School of Mines while working on a project for the National
% 	Renewable Energy Laboratory.
% It was further improved by Ali Hariri (research intern from CAPS-FSU) on June 6th, 2016. The code is made more consistent interms of
% 	terminology; more comments were added with references for better use in future work.
% It is based on the original bp_sx110 model created by Akihiro Oi (California Polytechnic State University) on 07/01/2005 
%	(see "Design and Simulation of Photovoltaic Water Pumping System" (September 2005)).
% Further PV model modifications were made based on the model presented in "Comprehensive Approach to Modeling and Simulation of 
% 	Photovoltaic Arrays" (2009) by Villalva et al.
% 
% Out:  Vout = array output voltage
%       Iout = Output current
%       VocMax = Open-Circuit Voltage
%       IscMax = Short-Circuit Current
% In:   Ns_module = Number of modules in series per string
%       Np_string = Number of strings in parallel
%       Tamb = ambient temperature in degrees celsius
%       G = Irradiance (1G = 1000 W/m^2) (can be input in W/m^2 or kW/m^2)
%       Vin = Voltage of load
%       Iout_old = Feedback loop from previous Iout

% *************************************************************************
%   Start Code
% *************************************************************************
Imeas = Imeas / 2;  % since we are using 5 modules of the magna power
                    % this code calculates the output for 1 

% if G is given in 1 W/m^2, convert to 1000 W/m^2
if G > 1.5
    G = G / 1000;
end

% Set all negative irradiances to 0
if G < 0
    G = 0;
end

% *************************************************************************
%   determine cell temperature from irradiance, windspeed, ambient temperature, and SAPM (sandia array performance model) module parameters
%		using King's SFP model (see pvl_sapmcelltemp): https://pvpmc.sandia.gov/PVLIB_Matlab_Help/html/pvl_sapmcelltemp_help.html
% *************************************************************************
G0 = 1000;                                          % reference irradiance type 1000 W/m2
windspeed = 10;                                     % use a default value for windspeed since its a second order effect
ap = -3.47;                                         % default for SAM glass/cell/glass
b = -0.0594;        %
deltaT = 3;         %
Tmodule = Tamb + (G*1000)*(exp(ap + b*windspeed));  % module temperature in degrees
Tcell_C = Tmodule + (G*1000/G0)*deltaT;				% cell temperature in degrees
Tcell_K = 273 + Tcell_C;                            % cell temperature in Kelvin

% *************************************************************************
%   Define and Calculate Constants and Variables
% *************************************************************************
% PV cell data
% ---------------------------------------------------------------------------------------
derating = 0.921;                                   % Panel derating factor
k = 1.381e-23;                                      % Boltzmanns constant
q = 1.602e-19;                                      % Electron charge
a = 1.25;                                           % Diode ideality factor (n),1 (ideal diode) < n < 2
Res = 400;                                          % I-V curve resolution - adjustable
Rs = 0.001;                                         % Series resistance per cell
Rp = 2;                                             % Parallel resistance per cell
TrK = 298;                                          % Reference temperature (25C) in Kelvin
Kv = -0.08;                                         % Voltage temperature coefficient (-80mV/C)
Ki = 0.65e-3;                                       % Temperature coefficient of Isc (0.065%/C)
% ---------------------------------------------------------------------------------------

% calculate module data
% ---------------------------------------------------------------------------------------
Ns_cell = 36*Ns_module;                               		% total number of series connected cells (BP SX110, 36 series cells per module)
Voc_TrK_module = 20.1;                                		% Voc in volts per module @ reference temp (V/panel)
Voc_TaK_module = Voc_TrK_module + (Kv*(Tcell_K - TrK));     % Voc per module @ actual temp
Voc = Voc_TaK_module/36;                              		% Voc per cell @ actual temp
Isc_nameplate = 7.38;                                 		% Isc per cell given on nameplate
Isc_TrK = Isc_nameplate*derating;                     		% Isc (short circuit current per cell) @ reference temp inclusive of derating
% ---------------------------------------------------------------------------------------

% *************************************************************************
%   Calculate outputs
% *************************************************************************

Isc = G *(Isc_TrK * (1 + (Ki * (Tcell_K - TrK))));      % Calculate PV cell short-circuit 'I' for given temp and irradiance
Vt =  k * Tcell_K / q;                                  % Define PV cell thermal potential (Vt) at actual temp
VocMax  = Voc_TaK_module*Ns_module;                     % max Voc per array due to temperature

% Set Vin to VocMax if requested Vin is beyond scope
if Vin > VocMax
    Vin = VocMax;
end
% ---------------------------------------------------------------------------------------

% If Vin is small, it is either startup or Isc.
% If it is Isc then Iout_old should be nearly Isc
if Vin < 1
    iTol = abs(Isc - (Iout_old/Np_string)) / (Iout_old/Np_string);
    % if Iout_old is within 5% of Isc
    if(iTol < 0.05)
        %use normal Vin value
    else
        %set Vout = Vin = Voc
        Vin = Ns_cell*Voc;
    end
end
% ---------------------------------------------------------------------------------------

Vc = Vin / Ns_cell;                                     	% Range of individual cell voltages of array
Io = Isc / (exp(Voc /(a* Vt)) -1);							% reverse saturation current for given temperature per cell
Id = (Io*(exp((Vc + (Iout_old/Np_string)*Rs)/(a*Vt))-1));  	% Diode + Series Resistance Current
Ip = (Vc + (Iout_old/Np_string)*Rs)/Rp;                    	% Parallel Resistance Current
Ia = Isc - Id - Ip;                            	% Final PV current (cell output)
% ---------------------------------------------------------------------------------------

% capture any negative commands to Ia out before they leave the block.
% This avoids negatives in the Ia delay feedback
% Ia1 = Np_string*Ia; % array output
if Ia < 0 
    Ia = 0;
end

IscMax = Isc*Np_string;
Vout = Vin;
% If Imeas is small (<10% of Isc) assume that we are at startup and set Iout = IscMax*0.3 
% (0.3 is chosen arbitrary smaller than Iscmax) otherwise use Ia
% if (Imeas <= 0.1 * IscMax)
%     Iout = IscMax * 0.3;
% else
%     Iout = Np_string*Ia;
% end
Iout = Np_string*Ia;
